simulink model "standalonewindturbine"  (R2024b)
settings: Solver=ode23tb  StartTime=0.0  StopTime=1  RelTol=1e-3  EnableMultiTasking=on
libraries: spsUniversalBridgeLib x2, spsThreePhaseVIMeasurementLib x1, spsWindTurbineLib x1, spsThreePhaseSeriesRLCLoadLib x1, spsParallelRLCBranchLib x1, spsSeriesRLCBranchLib x1, spsMeanLib x1, spsPWMGenerator2LevelLib x1, spsPermanentMagnetSynchronousMachineLib x1, spsRMSLib x1, powerlib_extras x1, spsVoltageMeasurementLib x1
settings Model: Creator=GOVIND  LastModifiedBy=realm
settings SolverCC: AlgebraicLoopSolver=TrustRegion
settings DataIOCC: LimitDataPoints=on  SaveFormat=Array  SignalLoggingSaveFormat=ModelDataLogs  ReturnWorkspaceOutputs=off
settings OptimizationCC: ExpressionDepthLimit=2147483647  LifeSpan=inf
settings DebuggingCC: UnderspecifiedInitializationDetection=Classic  MergeDetectMultiDrivingBlocksExec=none  FcnCallInpInsideContextMsg=warning  UnconnectedInputMsg=warning  UnconnectedOutputMsg=warning  UnconnectedLineMsg=warning  StateNameClashWarn=warning  SFUnexpectedBacktrackingDiag=warning  SFNoUnconditionalDefaultTransitionDiag=warning  SFExecutionAtInitializationDiag=none  ArithmeticOperatorsInVariantConditions=warning
settings HardwareCC: ProdBitPerPointer=32  ProdBitPerSizeT=32  ProdBitPerPtrDiffT=32  ProdLargestAtomicFloat=None  ProdIntDivRoundTo=Undefined  ProdEndianess=Unspecified  ProdWordSize=32  ProdHWDeviceType=32-bit Generic
settings ModelReferenceCC: EnableRefExpFcnMdlSchedulingChecks=on  PropagateSignalLabelsOutOfModel=off
settings SFSimCC: SimUseLocalCustomCode=off  CustomCodeUndefinedFunction=UseInterfaceOnly
settings RTWCC: RTWUseLocalCustomCode=off  GPUComputeCapability=3.5
settings CodeAppCC: StateflowObjectComments=on
settings GRTTargetCC: TargetLangStandard=C89/C90 (ANSI)  CombineOutputUpdateFcns=off  GRTInterface=on
settings ConfigComp: CovMetricSettings=dw  CovSaveCumulativeToWorkspaceVar=on  CovSaveSingleToWorkspaceVar=on  CovExternalEMLEnable=off

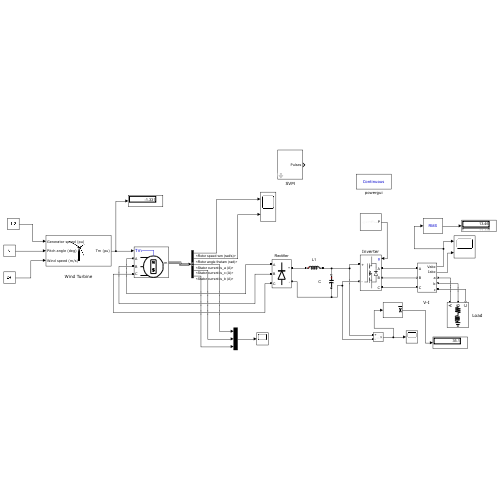
[thumbnail: Simulink's stored preview of the top-level diagram]
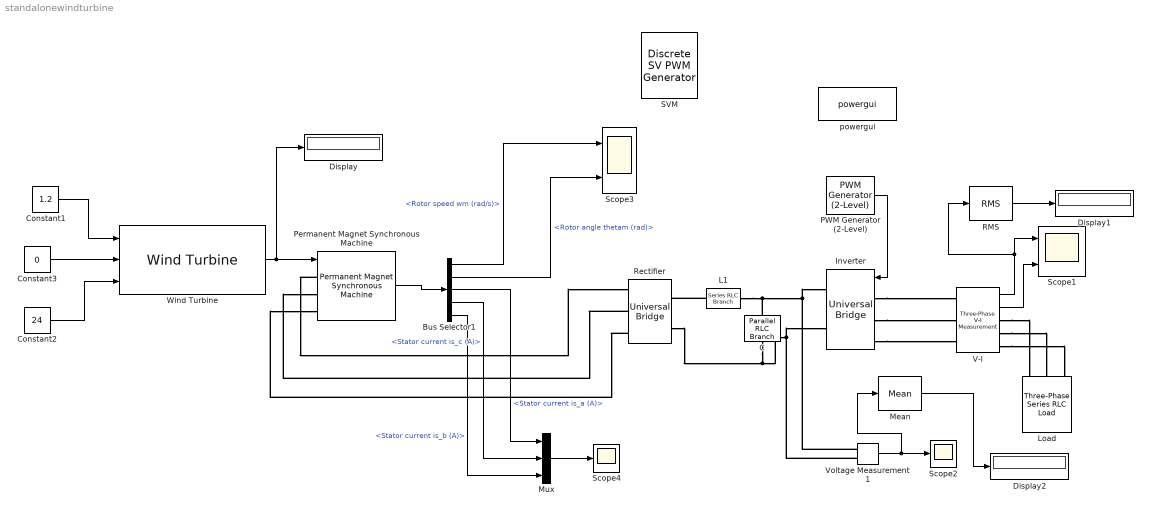
== system standalonewindturbine ==
  " V-I " : spsThreePhaseVIMeasurementLib/Three-Phase V-I Measurement  VoltageMeasurement=phase-to-ground  SetLabelV=off  LabelV=Vabc  Vpu=off  VpuLL=off  CurrentMeasurement=yes  SetLabelI=off  LabelI=Iabc  Ipu=off  Pbase=100e6  Vbase=500e3  OutputType=Complex  PhasorSimulation=off  PSBequivalent=0
  " Wind Turbine" : spsWindTurbineLib/Wind Turbine  Pnom=5000  Pelec_base=5000/0.9  wind_base=12  P_wind_base=0.73  speed_nom=1.2  pitch_angle=0  c1_c6="[0.51763          116          0.4            5           21     0.006795]"  cp_nom=0.48  lambda_nom=8.1
  " Load" : spsThreePhaseSeriesRLCLoadLib/Three-Phase Series RLC Load  LConnTagsString=A|B|C  Configuration=Y (grounded)  NominalVoltage=500  Vabc=[1e3 1e3 1e3]  Vabcp=[1e3 1e3 1e3]  NominalFrequency=50  UnbalancedPower=off  ActivePower=50000  InductivePower=100  CapacitivePower=0  Pabc=[10e3 9e3 11e3]  QLabc=[100 90 110]  QCabc=[100 90 110]  Pabcp=[10e3 9e3 11e3]  QLabcp=[100 90 110]  QCabcp=[100 90 110]  Measurements=None  LoadType=constant Z
  Bus Selector1 : BusSelector  OutputSignals=Rotor speed wm (rad/s),Rotor angle thetam (rad),Stator current is_a (A),Stator current is_c (A),Stator current is_b (A)
  C : spsParallelRLCBranchLib/Parallel RLC Branch  LConnTagsString=a  RConnTagsString=__new0  BranchType=C  Resistance=1.0  Inductance=1.0  SetiL0=off  InitialCurrent=0  Capacitance=5000e-06  Setx0=off  InitialVoltage=0  Measurements=None
  Constant1 : Constant  Value=1.2
  Constant2 : Constant  Value=24
  Constant3 : Constant  Value=0
  Display : Display
  Display1 : Display
  Display2 : Display
  Inverter : spsUniversalBridgeLib/Universal Bridge  Arms=3  SnubberResistance=1e5  SnubberCapacitance=inf  Device=MOSFET / Diodes  Ron=1e-3  Lon=0  ForwardVoltages="[  0  0  ]"  ForwardVoltage=0  GTOparameters=[ 10e-6 , 20e-6 ]  IGBTparameters=[ 1e-6 , 2e-6 ]  Measurements=None  Measurements_2=None  converterType=Rectifier
  L1 : spsSeriesRLCBranchLib/Series RLC Branch  LConnTagsString=__new0  RConnTagsString=__new0  BranchType=L  Resistance=1.0  Inductance=200e-6  SetiL0=off  InitialCurrent=0  Capacitance=1.0  Setx0=off  InitialVoltage=0  Measurements=None
  Mean : spsMeanLib/Mean  Freq=60  Vinit=0  Ts=0
  Mux : Mux  Inputs=3
  PWM Generator (2-Level) : spsPWMGenerator2LevelLib/PWM Generator (2-Level)  ModulatorType=Three-phase bridge (6 pulses)  ModulatorMode=Unsynchronized  Fc=1000  Pc=90  nF=27  MinMax="[ -1  1 ]"  SamplingTechnique=Natural  ModulatingSignals=on  m=0.8  Freq=50  Phase=0  Ts=0  ShowCarrierOutport=off
  Permanent Magnet Synchronous Machine : spsPermanentMagnetSynchronousMachineLib/Permanent Magnet Synchronous Machine  NbPhases=3  FluxDistribution=Sinusoidal  RotorType=Round  MechanicalLoad=Torque Tm  PresetModel="09:  7.14 Nm 560 Vdc 5000 RPM - 8.3 Nm"  ShowDetailedParameters=on  MeasurementBus=off  Resistance=0.24  Inductance=8.5e-3  dqInductances=[8.5e-3,8.5e-3]  La=0.001015  MachineConstant=Flux linkage established by magnets (V.s)  Flux=0.06784  VoltageCst=49.2193  TorqueCst=0.40704  Flat=120  Mechanical=[0.00048 0.0001619 4 0]  PolePairs=4  InitialConditions=[0,0, 0,0]  InitialConditions5ph=[0 0 0 0 0 0]  RefAngle=90 degrees behind phase A axis (modified Park)  IterativeDiscreteModel=Trapezoidal non iterative  TsBlock=-1  TsPowergui=0
  RMS : spsRMSLib/RMS  TrueRMS=on  Freq=50  RMSInit=120  Ts=0
  Rectifier : spsUniversalBridgeLib/Universal Bridge  Arms=3  SnubberResistance=100  SnubberCapacitance=0.1e-6  Device=Diodes  Ron=1e-3  Lon=0  ForwardVoltages="[  0.8  0.8  ]"  ForwardVoltage=.8  GTOparameters=[ 10e-6 , 20e-6 ]  IGBTparameters=[ 1e-6 , 2e-6 ]  Measurements=Device currents  Measurements_2=None  converterType=Rectifier
      settings: AttributesFormatString=\n
  SVM : powerlib_extras/Discrete  Control Blocks/Discrete SV PWM Generator  InputType=Internally generated  SwitchingPattern=Pattern #1  Fc=10000  ParUref=[0.9 0 50]  Ts=2e-6
  Scope1 : Scope  NumInputPorts=2
  Scope2 : Scope
  Scope3 : Scope  NumInputPorts=2
  Scope4 : Scope
  Voltage Measurement1 : spsVoltageMeasurementLib/Voltage Measurement  PhasorSimulation=off  OutputType=Complex  PSBequivalent=0
  powergui : spspowerguiLib/powergui  Priority=1  SimulationMode=Continuous  SampleTime=50e-6  frequency=50  Iterations=50  frequencyindice=0  Pbase=100e6  ErrMax=1e-4  UnitsV=kV  UnitsW=MW  buscounter=0  FunctionMessages=off  echomessages=off  EnableUseOfTLC=off  CurrentSourceSwitches=off  DisableSnubberDevices=off  DisableRonSwitches=off  DisableVfSwitches=off  DisplayEquations=off  AutomaticDiscreteSolvers=off  SolverType=Tustin/Backward Euler (TBE)  Interpol=off  ExternalGateDelay=off  methode=off  Ts=0  x0status=blocks  SPID=off  SwTol=0  HookPort=off  NonlinearTolerance=1e-4  nMaxIteration=100  ContinueOnMaxIteration=off  RestoreLinks=warning  ResistiveCurrentMeasurement=off  Frange=[0:2:500]  Ylog=off  Xlog=on  ShowGrid=off  save=off  variable=ZData  structure=simout2  ZoomFFT=on  StartTime=0.02  cycles=2  DisplayStyle=1  fundamental=50  FreqAxis=on  MaxFrequency=5000  frequencyindicesteady=1  RmsSteady=1  display=off
  wires:
  " V-I "/1 -> RMS/1, Scope1/1
  " V-I "/2 -> Scope1/2
  Permanent Magnet Synchronous Machine/1 -> Bus Selector1/1
  Constant3/1 -> " Wind Turbine"/2
  " Wind Turbine"/1 -> Display/1, Permanent Magnet Synchronous Machine/1
  Constant2/1 -> " Wind Turbine"/3
  Bus Selector1/1 -> Scope3/1  "<Rotor speed wm (rad/s)>"
  Bus Selector1/2 -> Scope3/2  "<Rotor angle thetam (rad)>"
  Constant1/1 -> " Wind Turbine"/1
  Voltage Measurement1/1 -> Mean/1, Scope2/1
  Bus Selector1/3 -> Mux/1  "<Stator current is_a (A)>"
  Bus Selector1/4 -> Mux/2  "<Stator current is_c (A)>"
  Bus Selector1/5 -> Mux/3  "<Stator current is_b (A)>"
  Mux/1 -> Scope4/1
  PWM Generator (2-Level)/1 -> Inverter/1
  RMS/1 -> Display1/1
  Mean/1 -> Display2/1
  connections:
  " V-I "/RConn1 -- " Load"/LConn1
  " V-I "/RConn2 -- " Load"/LConn2
  " V-I "/RConn3 -- " Load"/LConn3
  Rectifier/RConn2 -- C/RConn1 -- Voltage Measurement1/LConn2 -- Inverter/RConn2
  Rectifier/LConn2 -- Permanent Magnet Synchronous Machine/LConn2
  L1/RConn1 -- C/LConn1 -- Voltage Measurement1/LConn1 -- Inverter/RConn1
  Permanent Magnet Synchronous Machine/LConn1 -- Rectifier/LConn1
  Rectifier/LConn3 -- Permanent Magnet Synchronous Machine/LConn3
  L1/LConn1 -- Rectifier/RConn1
  Inverter/LConn1 -- " V-I "/LConn1
  Inverter/LConn2 -- " V-I "/LConn2
  Inverter/LConn3 -- " V-I "/LConn3
